simulink model "abs"  (Simulink 6.6)
settings: Solver=FixedStepDiscrete  StartTime=0.0  StopTime=10.0  FixedStep=1  RelTol=1e-3
settings Model: Creator=ksmyth  LastModifiedBy=ksmyth

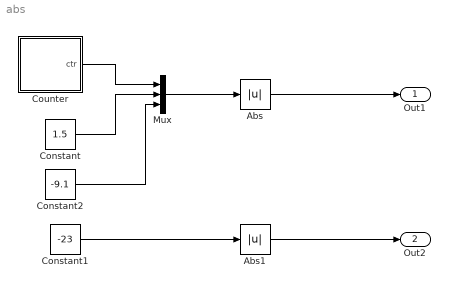
== system abs ==
  Abs : Abs
  Abs1 : Abs
  Constant : Constant  Value=1.5
  Constant1 : Constant  Value=-23
  Constant2 : Constant  Value=-9.1
  Counter : Stateflow chart
  Mux : Mux  Inputs=3
  Out1 : Outport
  Out2 : Outport  Port=2
  wires:
  Counter/1(ctr) -> Mux/1
  Mux/1 -> Abs/1
  Abs/1 -> Out1/1
  Constant/1 -> Mux/2
  Constant1/1 -> Abs1/1
  Abs1/1 -> Out2/1
  Constant2/1 -> Mux/3

== stateflow chart Counter ==
  state s1
  (default) -> s1
  s1 -> s1 [order 1] : [ctr < 4] / ctr = ctr+1;
  s1 -> s1 [order 2] : [ctr >= 4] / ctr = -2;
  data: ctr output double =1
